simulink model "Simulation"  (R2025a)
settings: Solver=VariableStepAuto  StartTime=0.0  StopTime=10.0  RelTol=1e-3
libraries: simulink x6, simulink_extras x2
settings Model: Creator=Janik  LastModifiedBy=Janik

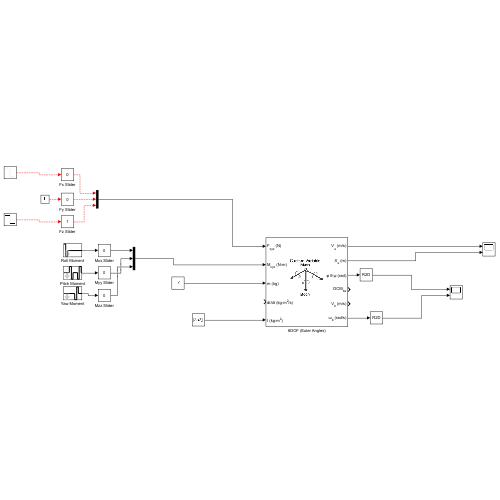
[thumbnail: Simulink's stored preview of the top-level diagram]
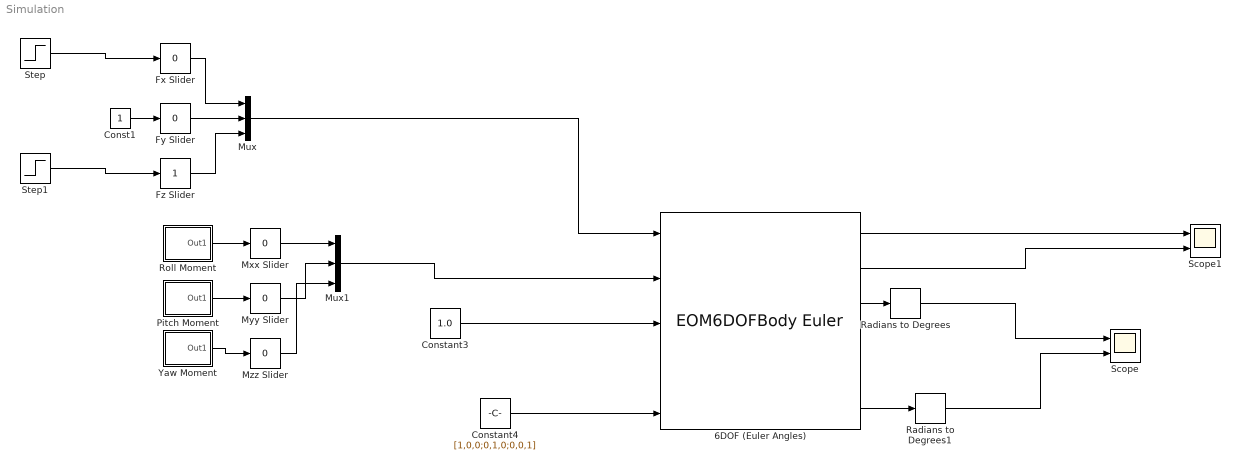
== system Simulation ==
  6DOF (Euler Angles) : EOM6DOFBodyEuler  mtype=Custom Variable  mass_flag=on
  Const1 : Constant
  Constant3 : Constant  Value=1.0
  Constant4 : Constant  Value=[1,0,0;0,1,0;0,0,1]  VectorParams1D=off
  Fx Slider : simulink/Math Operations/Slider Gain  gain=0  low=-1  high=1
  Fy Slider : simulink/Math Operations/Slider Gain  gain=0  low=-1  high=1
  Fz Slider : simulink/Math Operations/Slider Gain  gain=1  low=-1  high=1
  Mux : Mux  Inputs=3
  Mux1 : Mux  Inputs=3
  Mxx Slider : simulink/Math Operations/Slider Gain  gain=0  low=-5  high=10
  Myy Slider : simulink/Math Operations/Slider Gain  gain=0  low=-10  high=10
  Mzz Slider : simulink/Math Operations/Slider Gain  gain=0  low=-1  high=1
  Pitch Moment : Subsystem  mask(timed input){t=[0 3 3 4 4 5 5  7.5 7.5 8.5 8.5 9.5 9.5 10], u=[0 0  1 1 -1 -1.005 0 0 -1 -1 1 1 0 0]*3.138/2}
      mask prompts: t "time values:"; u "input values"
      mask Display: plot(t,u)
  Radians to Degrees : simulink_extras/Transformations/Radians to Degrees
  Radians to Degrees1 : simulink_extras/Transformations/Radians to Degrees
  Roll Moment : Subsystem  mask(timed input){t=[0 1 1 2 2  10], u=[1 1 -1 -.998  0 0]*3.144/2}
      mask prompts: t "time values:"; u "input values"
      mask Display: plot(t,u)
  Scope : Scope  NumInputPorts=2
      settings: ActiveDisplayYMinimum=-294.78665616471727  ActiveDisplayYMaximum=306.73025806988079
  Scope1 : Scope  NumInputPorts=2
      settings: ActiveDisplayYMinimum=-75.638957803935469  ActiveDisplayYMaximum=119.61899282163635
  Step : Step  Before=10  After=0  SampleTime=0
  Step1 : Step  Before=10  After=0  SampleTime=0
  Yaw Moment : Subsystem  mask(timed input){t=[0 6 6 7 7 8 8 10], u=[0 0  -1 -1 1 1 0 0]*3.1/2}
      mask prompts: t "time values:"; u "input values"
      mask Display: plot(t,u)
  wires:
  Constant3/1 -> 6DOF (Euler Angles)/3
  Constant4/1 -> 6DOF (Euler Angles)/5
  Fx Slider/1 -> Mux/1
  Fy Slider/1 -> Mux/2
  Step/1 -> Fx Slider/1
  Fz Slider/1 -> Mux/3
  Step1/1 -> Fz Slider/1
  Const1/1 -> Fy Slider/1
  Mxx Slider/1 -> Mux1/1
  Mzz Slider/1 -> Mux1/3
  Yaw Moment/1(Out1) -> Mzz Slider/1
  Pitch Moment/1(Out1) -> Myy Slider/1
  Myy Slider/1 -> Mux1/2
  Roll Moment/1(Out1) -> Mxx Slider/1
  Mux/1 -> 6DOF (Euler Angles)/1
  Mux1/1 -> 6DOF (Euler Angles)/2
  6DOF (Euler Angles)/1 -> Scope1/1
  6DOF (Euler Angles)/2 -> Scope1/2
  6DOF (Euler Angles)/3 -> Radians to Degrees/1
  6DOF (Euler Angles)/6 -> Radians to Degrees1/1
  Radians to Degrees1/1 -> Scope/2
  Radians to Degrees/1 -> Scope/1

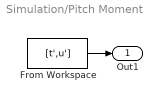
== system Simulation/Pitch Moment ==
  From Workspace : FromWorkspace  VariableName=[t',u']  ZeroCross=off
  Out1 : Outport  InitialOutput=0  VectorParamsAs1DForOutWhenUnconnected=off
  wires:
  From Workspace/1 -> Out1/1

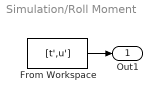
== system Simulation/Roll Moment ==
  From Workspace : FromWorkspace  VariableName=[t',u']  ZeroCross=off
  Out1 : Outport  InitialOutput=0  VectorParamsAs1DForOutWhenUnconnected=off
  wires:
  From Workspace/1 -> Out1/1

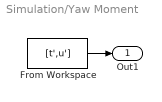
== system Simulation/Yaw Moment ==
  From Workspace : FromWorkspace  VariableName=[t',u']  ZeroCross=off
  Out1 : Outport  InitialOutput=0  VectorParamsAs1DForOutWhenUnconnected=off
  wires:
  From Workspace/1 -> Out1/1
